simulink model "lc_state_fb_obs_estStatesR"  (R2019a)
settings: Solver=VariableStepAuto  StartTime=0.0  StopTime=60  RelTol=1e-3
values from neighbouring files (symbols this model uses):
  A = [-2 -timeHeadway 0]    [Controller.m]    (also in SimulinkScenario.m = [1 0 0;beta1 1 0; beta0 beta1 1; 0 beta0 beta1; 0 0 beta0])
  B = [0; b1; 0; b2]    [SimulinkScenario.m]
  C = [1 timeHeadway 0; 0 1 timeHeadway; 0 0 1]    [Controller.m]    (also in SimulinkScenario.m = [1 0 0 0])
  Cf = 12e3    (= 12000)    [sim_parameters.m]
  Cr = 11e3    (= 11000)    [sim_parameters.m]
  Iz = 4000    [sim_parameters.m]
  K = A\z    [SimulinkScenario.m]
  L = place(A', C', poles*3)'    [SimulinkScenario.m]
  lf = 1.4    [sim_parameters.m]
  lr = 1.6    [sim_parameters.m]
  maxDelta = 25*pi/180    (= 0.436332312999)    [sim_parameters.m]
  maxDeltaDot = 9.4*pi/180    (= 0.164060949687)    [sim_parameters.m]
  vehMass = 2000    [sim_parameters.m]
  vxRef = 20    [SimulinkScenario.m]
libraries: dspsigops x5, autolibshared x5
settings Model: Creator=Fernando VM  LastModifiedBy=fvall

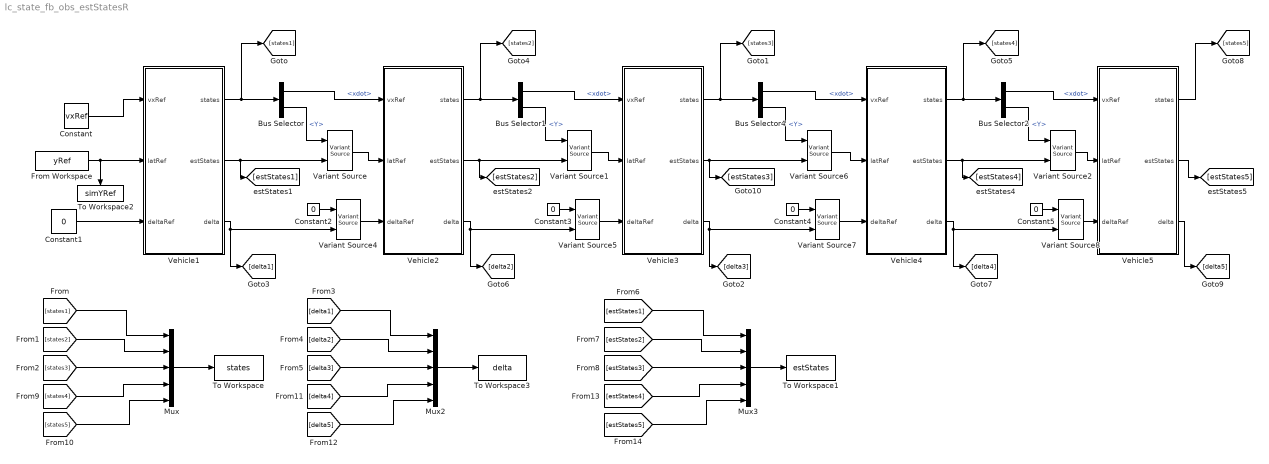
== system lc_state_fb_obs_estStatesR ==
  Bus Selector{,1..2,4} (4 alike) : BusSelector  OutputSignals=xdot,Y
  Constant : Constant  Value=vxRef
  Constant{1..5} (5 alike) : Constant  Value=0
  From Workspace : FromWorkspace  VariableName=yRef  SampleTime=0
  Mux : Mux  Inputs=5
  Mux2 : Mux  Inputs=5
  Mux3 : Mux  Inputs=5
  To Workspace : ToWorkspace  VariableName=states  SampleTime=-1
  To Workspace1 : ToWorkspace  VariableName=estStates  SampleTime=-1
  To Workspace2 : ToWorkspace  VariableName=simYRef  SampleTime=-1
  To Workspace3 : ToWorkspace  VariableName=delta  SampleTime=-1
  Variant Source{,1..2,4..8} (8 alike) : VariantSource
  Vehicle1 : Subsystem  mask{maxDelta=maxDelta, maxDeltaDot=maxDeltaDot, m=vehMass, a=lf, b=lr, Cy_f=Cr, Cy_r=Cf, Izz=Iz, X_o=38.84, initVel=20, sysMatrix=A, inputMatrix=B, C=C, feedbackGain=K, observerGain=L, inputTau=0}
      mask prompts: maxDelta "Max Delta"; maxDeltaDot "Max Delta Variation"; m "autoblks_shared:autoblkVehBody3DofLat:blkPrm_m"; a "autoblks_shared:autoblkVehBody3DofLat:blkPrm_a"; b "autoblks_shared:autoblkVehBody3DofLat:blkPrm_b"; Cy_f "autoblks_shared:autoblkVehBody3DofLat:blkPrm_Cy_f"; Cy_r "autoblks_shared:autoblkVehBody3DofLat:blkPrm_Cy_r"; Izz "autoblks_shared:autoblkVehBody3DofLat:blkPrm_Izz"; X_o "autoblks_shared:autoblkVehBody3DofLat:blkPrm_X_o"; initVel "Initial Long Velocity"; sysMatrix "A"; inputMatrix "B"; feedbackGain "State Feedback Gain Vector"; observerGain "Observer Gain"; inputTau "Input filter time constant"
      mask TypeOptions m: Vehicle Body 3DOF Single Track/m
      mask TypeOptions a: Vehicle Body 3DOF Single Track/a
      mask TypeOptions b: Vehicle Body 3DOF Single Track/b
      mask TypeOptions Cy_f: Vehicle Body 3DOF Single Track/Cy_f
      mask TypeOptions Cy_r: Vehicle Body 3DOF Single Track/Cy_r
      mask TypeOptions Izz: Vehicle Body 3DOF Single Track/Izz
      mask TypeOptions X_o: Vehicle Body 3DOF Single Track/X_o
      mask DialogControl ParameterGroupVar Prompt: Vehicle Parameters
      mask DialogControl m Prompt: Vehicle mass, m [kg]:
      mask DialogControl a Prompt: Longitudinal distance from center of mass to front axle, a [m]:
      mask DialogControl b Prompt: Longitudinal distance from center of mass to rear axle, b [m]:
      mask DialogControl Cy_f Prompt: Front tire corner stiffness, Cy_f [N/rad]:
      mask DialogControl Cy_r Prompt: Rear tire axle corner stiffness, Cy_r [N/rad]:
      mask DialogControl Izz Prompt: Yaw polar inertia, Izz [kg*m^2]:
      mask DialogControl Container6 Prompt: Initial Conditions
      mask DialogControl X_o Prompt: Initial inertial frame longitudinal position, X_o [m]:
      mask DialogControl Container3 Prompt: Linear Model
      mask DialogControl Container5 Prompt: Controller
  Vehicle2 : Subsystem  mask{maxDelta=maxDelta, maxDeltaDot=maxDeltaDot, m=vehMass, a=lf, b=lr, Cy_f=Cr, Cy_r=Cf, Izz=Iz, X_o=29.13, initVel=20, sysMatrix=A, inputMatrix=B, C=C, feedbackGain=K, observerGain=L, inputTau=0}
      mask prompts: maxDelta "Max Delta"; maxDeltaDot "Max Delta Variation"; m "autoblks_shared:autoblkVehBody3DofLat:blkPrm_m"; a "autoblks_shared:autoblkVehBody3DofLat:blkPrm_a"; b "autoblks_shared:autoblkVehBody3DofLat:blkPrm_b"; Cy_f "autoblks_shared:autoblkVehBody3DofLat:blkPrm_Cy_f"; Cy_r "autoblks_shared:autoblkVehBody3DofLat:blkPrm_Cy_r"; Izz "autoblks_shared:autoblkVehBody3DofLat:blkPrm_Izz"; X_o "autoblks_shared:autoblkVehBody3DofLat:blkPrm_X_o"; initVel "Initial Long Velocity"; sysMatrix "A"; inputMatrix "B"; feedbackGain "State Feedback Gain Vector"; observerGain "Observer Gain"; inputTau "Input filter time constant"
      mask TypeOptions m: Vehicle Body 3DOF Single Track/m
      mask TypeOptions a: Vehicle Body 3DOF Single Track/a
      mask TypeOptions b: Vehicle Body 3DOF Single Track/b
      mask TypeOptions Cy_f: Vehicle Body 3DOF Single Track/Cy_f
      mask TypeOptions Cy_r: Vehicle Body 3DOF Single Track/Cy_r
      mask TypeOptions Izz: Vehicle Body 3DOF Single Track/Izz
      mask TypeOptions X_o: Vehicle Body 3DOF Single Track/X_o
      mask DialogControl ParameterGroupVar Prompt: Vehicle Parameters
      mask DialogControl m Prompt: Vehicle mass, m [kg]:
      mask DialogControl a Prompt: Longitudinal distance from center of mass to front axle, a [m]:
      mask DialogControl b Prompt: Longitudinal distance from center of mass to rear axle, b [m]:
      mask DialogControl Cy_f Prompt: Front tire corner stiffness, Cy_f [N/rad]:
      mask DialogControl Cy_r Prompt: Rear tire axle corner stiffness, Cy_r [N/rad]:
      mask DialogControl Izz Prompt: Yaw polar inertia, Izz [kg*m^2]:
      mask DialogControl Container6 Prompt: Initial Conditions
      mask DialogControl X_o Prompt: Initial inertial frame longitudinal position, X_o [m]:
      mask DialogControl Container3 Prompt: Linear Model
      mask DialogControl Container5 Prompt: Controller
  Vehicle3 : Subsystem  mask{maxDelta=maxDelta, maxDeltaDot=maxDeltaDot, m=vehMass, a=lf, b=lr, Cy_f=Cr, Cy_r=Cf, Izz=Iz, X_o=19.42, initVel=20, sysMatrix=A, inputMatrix=B, C=C, feedbackGain=K, observerGain=L, inputTau=0}
      mask prompts: maxDelta "Max Delta"; maxDeltaDot "Max Delta Variation"; m "autoblks_shared:autoblkVehBody3DofLat:blkPrm_m"; a "autoblks_shared:autoblkVehBody3DofLat:blkPrm_a"; b "autoblks_shared:autoblkVehBody3DofLat:blkPrm_b"; Cy_f "autoblks_shared:autoblkVehBody3DofLat:blkPrm_Cy_f"; Cy_r "autoblks_shared:autoblkVehBody3DofLat:blkPrm_Cy_r"; Izz "autoblks_shared:autoblkVehBody3DofLat:blkPrm_Izz"; X_o "autoblks_shared:autoblkVehBody3DofLat:blkPrm_X_o"; initVel "Initial Long Velocity"; sysMatrix "A"; inputMatrix "B"; feedbackGain "State Feedback Gain Vector"; observerGain "Observer Gain"; inputTau "Input filter time constant"
      mask TypeOptions m: Vehicle Body 3DOF Single Track/m
      mask TypeOptions a: Vehicle Body 3DOF Single Track/a
      mask TypeOptions b: Vehicle Body 3DOF Single Track/b
      mask TypeOptions Cy_f: Vehicle Body 3DOF Single Track/Cy_f
      mask TypeOptions Cy_r: Vehicle Body 3DOF Single Track/Cy_r
      mask TypeOptions Izz: Vehicle Body 3DOF Single Track/Izz
      mask TypeOptions X_o: Vehicle Body 3DOF Single Track/X_o
      mask DialogControl ParameterGroupVar Prompt: Vehicle Parameters
      mask DialogControl m Prompt: Vehicle mass, m [kg]:
      mask DialogControl a Prompt: Longitudinal distance from center of mass to front axle, a [m]:
      mask DialogControl b Prompt: Longitudinal distance from center of mass to rear axle, b [m]:
      mask DialogControl Cy_f Prompt: Front tire corner stiffness, Cy_f [N/rad]:
      mask DialogControl Cy_r Prompt: Rear tire axle corner stiffness, Cy_r [N/rad]:
      mask DialogControl Izz Prompt: Yaw polar inertia, Izz [kg*m^2]:
      mask DialogControl Container6 Prompt: Initial Conditions
      mask DialogControl X_o Prompt: Initial inertial frame longitudinal position, X_o [m]:
      mask DialogControl Container3 Prompt: Linear Model
      mask DialogControl Container5 Prompt: Controller
  Vehicle4 : Subsystem  mask{maxDelta=maxDelta, maxDeltaDot=maxDeltaDot, m=vehMass, a=lf, b=lr, Cy_f=Cr, Cy_r=Cf, Izz=Iz, X_o=9.71, initVel=20, sysMatrix=A, inputMatrix=B, C=C, feedbackGain=K, observerGain=L, inputTau=0}
      mask prompts: maxDelta "Max Delta"; maxDeltaDot "Max Delta Variation"; m "autoblks_shared:autoblkVehBody3DofLat:blkPrm_m"; a "autoblks_shared:autoblkVehBody3DofLat:blkPrm_a"; b "autoblks_shared:autoblkVehBody3DofLat:blkPrm_b"; Cy_f "autoblks_shared:autoblkVehBody3DofLat:blkPrm_Cy_f"; Cy_r "autoblks_shared:autoblkVehBody3DofLat:blkPrm_Cy_r"; Izz "autoblks_shared:autoblkVehBody3DofLat:blkPrm_Izz"; X_o "autoblks_shared:autoblkVehBody3DofLat:blkPrm_X_o"; initVel "Initial Long Velocity"; sysMatrix "A"; inputMatrix "B"; feedbackGain "State Feedback Gain Vector"; observerGain "Observer Gain"; inputTau "Input filter time constant"
      mask TypeOptions m: Vehicle Body 3DOF Single Track/m
      mask TypeOptions a: Vehicle Body 3DOF Single Track/a
      mask TypeOptions b: Vehicle Body 3DOF Single Track/b
      mask TypeOptions Cy_f: Vehicle Body 3DOF Single Track/Cy_f
      mask TypeOptions Cy_r: Vehicle Body 3DOF Single Track/Cy_r
      mask TypeOptions Izz: Vehicle Body 3DOF Single Track/Izz
      mask TypeOptions X_o: Vehicle Body 3DOF Single Track/X_o
      mask DialogControl ParameterGroupVar Prompt: Vehicle Parameters
      mask DialogControl m Prompt: Vehicle mass, m [kg]:
      mask DialogControl a Prompt: Longitudinal distance from center of mass to front axle, a [m]:
      mask DialogControl b Prompt: Longitudinal distance from center of mass to rear axle, b [m]:
      mask DialogControl Cy_f Prompt: Front tire corner stiffness, Cy_f [N/rad]:
      mask DialogControl Cy_r Prompt: Rear tire axle corner stiffness, Cy_r [N/rad]:
      mask DialogControl Izz Prompt: Yaw polar inertia, Izz [kg*m^2]:
      mask DialogControl Container6 Prompt: Initial Conditions
      mask DialogControl X_o Prompt: Initial inertial frame longitudinal position, X_o [m]:
      mask DialogControl Container3 Prompt: Linear Model
      mask DialogControl Container5 Prompt: Controller
  Vehicle5 : Subsystem  mask{maxDelta=maxDelta, maxDeltaDot=maxDeltaDot, m=vehMass, a=lf, b=lr, Cy_f=Cr, Cy_r=Cf, Izz=Iz, X_o=0, initVel=20, sysMatrix=A, inputMatrix=B, C=C, feedbackGain=K, observerGain=L, inputTau=0}
      mask prompts: maxDelta "Max Delta"; maxDeltaDot "Max Delta Variation"; m "autoblks_shared:autoblkVehBody3DofLat:blkPrm_m"; a "autoblks_shared:autoblkVehBody3DofLat:blkPrm_a"; b "autoblks_shared:autoblkVehBody3DofLat:blkPrm_b"; Cy_f "autoblks_shared:autoblkVehBody3DofLat:blkPrm_Cy_f"; Cy_r "autoblks_shared:autoblkVehBody3DofLat:blkPrm_Cy_r"; Izz "autoblks_shared:autoblkVehBody3DofLat:blkPrm_Izz"; X_o "autoblks_shared:autoblkVehBody3DofLat:blkPrm_X_o"; initVel "Initial Long Velocity"; sysMatrix "A"; inputMatrix "B"; feedbackGain "State Feedback Gain Vector"; observerGain "Observer Gain"; inputTau "Input filter time constant"
      mask TypeOptions m: Vehicle Body 3DOF Single Track/m
      mask TypeOptions a: Vehicle Body 3DOF Single Track/a
      mask TypeOptions b: Vehicle Body 3DOF Single Track/b
      mask TypeOptions Cy_f: Vehicle Body 3DOF Single Track/Cy_f
      mask TypeOptions Cy_r: Vehicle Body 3DOF Single Track/Cy_r
      mask TypeOptions Izz: Vehicle Body 3DOF Single Track/Izz
      mask TypeOptions X_o: Vehicle Body 3DOF Single Track/X_o
      mask DialogControl ParameterGroupVar Prompt: Vehicle Parameters
      mask DialogControl m Prompt: Vehicle mass, m [kg]:
      mask DialogControl a Prompt: Longitudinal distance from center of mass to front axle, a [m]:
      mask DialogControl b Prompt: Longitudinal distance from center of mass to rear axle, b [m]:
      mask DialogControl Cy_f Prompt: Front tire corner stiffness, Cy_f [N/rad]:
      mask DialogControl Cy_r Prompt: Rear tire axle corner stiffness, Cy_r [N/rad]:
      mask DialogControl Izz Prompt: Yaw polar inertia, Izz [kg*m^2]:
      mask DialogControl Container6 Prompt: Initial Conditions
      mask DialogControl X_o Prompt: Initial inertial frame longitudinal position, X_o [m]:
      mask DialogControl Container3 Prompt: Linear Model
      mask DialogControl Container5 Prompt: Controller
  wires:
  From Workspace/1 -> Vehicle1/2(latRef), To Workspace2/1
  Constant/1 -> Vehicle1/1(vxRef)
  Vehicle1/1(states) -> [states1], Bus Selector/1
  Vehicle1/2(estStates) -> [estStates1], Variant Source/2
  Mux/1 -> To Workspace/1
  [states1] -> Mux/1
  [states2] -> Mux/2
  [states3] -> Mux/3
  Vehicle1/3(delta) -> [delta1], Variant Source4/2
  [states4] -> Mux/4
  [states5] -> Mux/5
  [delta4] -> Mux2/4
  [delta5] -> Mux2/5
  [delta1] -> Mux2/1
  [delta2] -> Mux2/2
  [delta3] -> Mux2/3
  Mux2/1 -> To Workspace3/1
  [estStates4] -> Mux3/4
  [estStates5] -> Mux3/5
  [estStates1] -> Mux3/1
  [estStates2] -> Mux3/2
  [estStates3] -> Mux3/3
  Mux3/1 -> To Workspace1/1
  Bus Selector/2 -> Variant Source/1  "<Y>"
  Bus Selector/1 -> Vehicle2/1(vxRef)  "<xdot>"
  Variant Source/1 -> Vehicle2/2(latRef)
  Constant1/1 -> Vehicle1/3(deltaRef)
  Constant2/1 -> Variant Source4/1
  Variant Source4/1 -> Vehicle2/3(deltaRef)
  Bus Selector1/2 -> Variant Source1/1  "<Y>"
  Vehicle2/2(estStates) -> [estStates2], Variant Source1/2
  Vehicle2/3(delta) -> [delta2], Variant Source5/2
  Variant Source5/1 -> Vehicle3/3(deltaRef)
  Vehicle2/1(states) -> [states2], Bus Selector1/1
  Bus Selector1/1 -> Vehicle3/1(vxRef)  "<xdot>"
  Variant Source1/1 -> Vehicle3/2(latRef)
  Constant3/1 -> Variant Source5/1
  Constant4/1 -> Variant Source7/1
  Vehicle3/2(estStates) -> Variant Source6/2, [estStates3]
  Bus Selector4/2 -> Variant Source6/1  "<Y>"
  Vehicle3/3(delta) -> [delta3], Variant Source7/2
  Vehicle3/1(states) -> [states3], Bus Selector4/1
  Constant5/1 -> Variant Source8/1
  Vehicle4/2(estStates) -> [estStates4], Variant Source2/2
  Bus Selector2/2 -> Variant Source2/1  "<Y>"
  Vehicle4/3(delta) -> [delta4], Variant Source8/2
  Vehicle4/1(states) -> [states4], Bus Selector2/1
  Variant Source7/1 -> Vehicle4/3(deltaRef)
  Variant Source6/1 -> Vehicle4/2(latRef)
  Vehicle5/2(estStates) -> [estStates5]
  Vehicle5/3(delta) -> [delta5]
  Vehicle5/1(states) -> [states5]
  Variant Source8/1 -> Vehicle5/3(deltaRef)
  Variant Source2/1 -> Vehicle5/2(latRef)
  Bus Selector2/1 -> Vehicle5/1(vxRef)  "<xdot>"
  Bus Selector4/1 -> Vehicle4/1(vxRef)  "<xdot>"

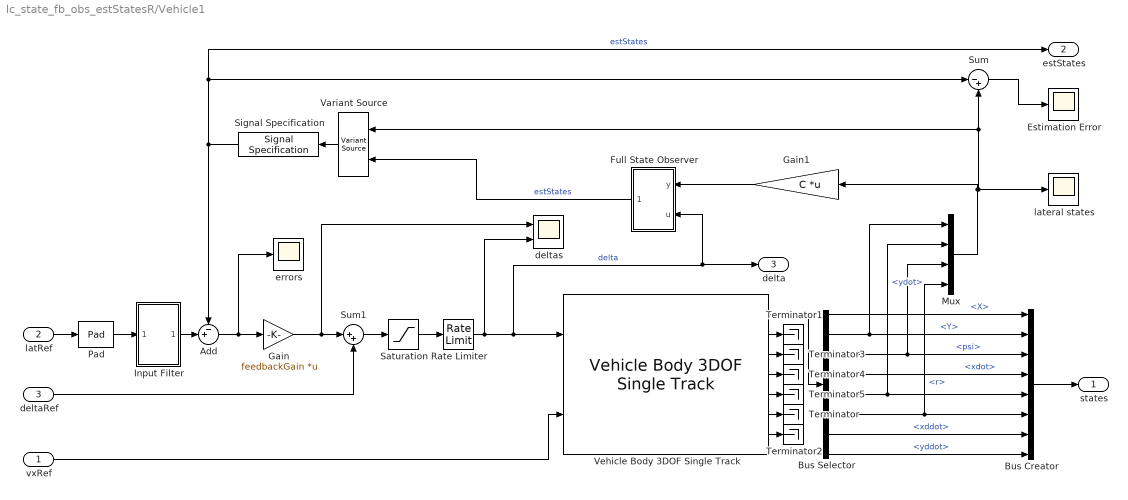
== system lc_state_fb_obs_estStatesR/Vehicle1 ==
  vxRef : Inport
  latRef : Inport  Port=2
  deltaRef : Inport  Port=3
  Add : Sum  Inputs=-+|
  Bus Creator : BusCreator  Inputs=8
  Bus Selector : BusSelector  OutputSignals=InertFrm.Cg.Disp.X,InertFrm.Cg.Disp.Y,InertFrm.Cg.Ang.psi,BdyFrm.Cg.Vel.xdot,BdyFrm.Cg.Vel.ydot,BdyFrm.Cg.AngVel.r,BdyFrm.Cg.Acc.xddot,BdyFrm.Cg.Acc.yddot
  Estimation Error : Scope
  Full State Observer : Subsystem
  Gain : Gain  Gain=feedbackGain  Multiplication=Matrix(K*u)
  Gain1 : Gain  Gain=C  Multiplication=Matrix(K*u)
  Input Filter : Subsystem
  Mux : Mux
  Pad : dspsigops/Pad  padAlong=Columns  dimsToPad=1  valSrc=Specify via dialog  padVal=0  spec=Output size  padNumOutRowsSpecMethod=User-specified  numOutRows=4  padNumOutColsSpecMethod=User-specified  numOutCols=1  isVarDimsMode=off  padBeginning=0  padEnd=0  outSizeMode=User-specified  outSize=1  padSigAt=End  trunc_flag=None  roundingMode=Floor  overflowMode=off  truncOrWrapMode=Truncate  wrap_flag=None
      settings: SourceProductName=DSP System Toolbox  SourceProductBaseCode=DS
  Rate Limiter : RateLimiter  RisingSlewLimit=maxDeltaDot  FallingSlewLimit=-maxDeltaDot  SampleTimeMode=inherited
  Saturation : Saturate  UpperLimit=maxDelta  LowerLimit=-maxDelta
  Signal Specification : SignalSpecification  Dimensions=[4 1]
  Sum : Sum  Inputs=|-+
  Sum1 : Sum  Inputs=|++
  Terminator{,1..5} (6 alike) : Terminator
  Variant Source : VariantSource
  Vehicle Body 3DOF Single Track : autolibshared/Vehicle Body 3DOF Single Track  trackMode=Single (bicycle)  inputMode=External longitudinal velocity  frontSteerMode=on  rearSteerMode=off  windMode=off  muMode=off  extFMode=off  extMMode=off  extXo=off  extpsio=off  extxdoto=off  extro=off  extYo=off  extTamb=off  extydoto=off  aMode=2  NF=2  NR=2  m=m  a=a  b=b  h=0.35  X_o=X_o  xdot_o=0  CalphaMode=off  sigmaMode=on  d=0  w=[1.4,1.4]  Cy_f=Cy_f  Cy_r=Cy_r  sigma_f=.1  sigma_r=.1  alpha_f_brk=[-.1 .1]  Cy_f_data=[-9e3 9e3]  alpha_r_brk=[-.1 .1]  Cy_r_data=[-9e3 9e3]  Y_o=0  ydot_o=0  Izz=Izz  psi_o=0  r_o=0  Af=2  Cd=.3  Cl=.1  Cpm=.1  beta_w=[0:0.01:0.3]  Cs=[0:0.03:0.9]  Cym=[0:0.01:0.3]  Pabs=101325  Tair=273  g=9.81  mu=1  xdot_tol=.01  Fznom=5000  Fxtire_sat=7e4  Fytire_sat=7e4  longOff=0  latOff=0  vertOff=0  wrapAng=off
      settings: SourceProductName=Powertrain Blockset  SourceProductBaseCode=PW
  deltas : Scope  NumInputPorts=2
  errors : Scope
  lateral states : Scope
  states : Outport
  estStates : Outport  Port=2
  delta : Outport  Port=3
  wires:
  Add/1 -> errors/1, Gain/1
  Gain/1 -> Sum1/1, deltas/1
  Vehicle Body 3DOF Single Track/1 -> Bus Selector/1
  Bus Selector/2 -> Bus Creator/2, Mux/1  "<Y>"
  Saturation/1 -> Rate Limiter/1
  vxRef/1 -> Vehicle Body 3DOF Single Track/2
  Sum/1 -> Estimation Error/1
  latRef/1 -> Pad/1
  Input Filter/1(Out1) -> Add/2
  Vehicle Body 3DOF Single Track/2 -> Terminator1/1
  Vehicle Body 3DOF Single Track/6 -> Terminator/1
  Vehicle Body 3DOF Single Track/7 -> Terminator2/1
  Bus Selector/5 -> Mux/2, Bus Creator/5  "<ydot>"
  Bus Selector/3 -> Bus Creator/3, Mux/3  "<psi>"
  Bus Selector/6 -> Bus Creator/6, Mux/4  "<r>"
  Vehicle Body 3DOF Single Track/3 -> Terminator3/1
  Vehicle Body 3DOF Single Track/4 -> Terminator4/1
  Vehicle Body 3DOF Single Track/5 -> Terminator5/1
  Bus Creator/1 -> states/1
  Bus Selector/1 -> Bus Creator/1  "<X>"
  Bus Selector/4 -> Bus Creator/4  "<xdot>"
  Bus Selector/7 -> Bus Creator/7  "<xddot>"
  Bus Selector/8 -> Bus Creator/8  "<yddot>"
  Variant Source/1 -> Signal Specification/1
  Gain1/1 -> Full State Observer/1(y)
  Mux/1 -> Gain1/1, Variant Source/1, Sum/2, lateral states/1
  Full State Observer/1(xhat) -> Variant Source/2  "estStates"
  Rate Limiter/1 -> Vehicle Body 3DOF Single Track/1, Full State Observer/2(u), delta/1, deltas/2  "delta"
  Signal Specification/1 -> estStates/1, Sum/1, Add/1  "estStates"
  Pad/1 -> Input Filter/1(In1)
  Sum1/1 -> Saturation/1
  deltaRef/1 -> Sum1/2

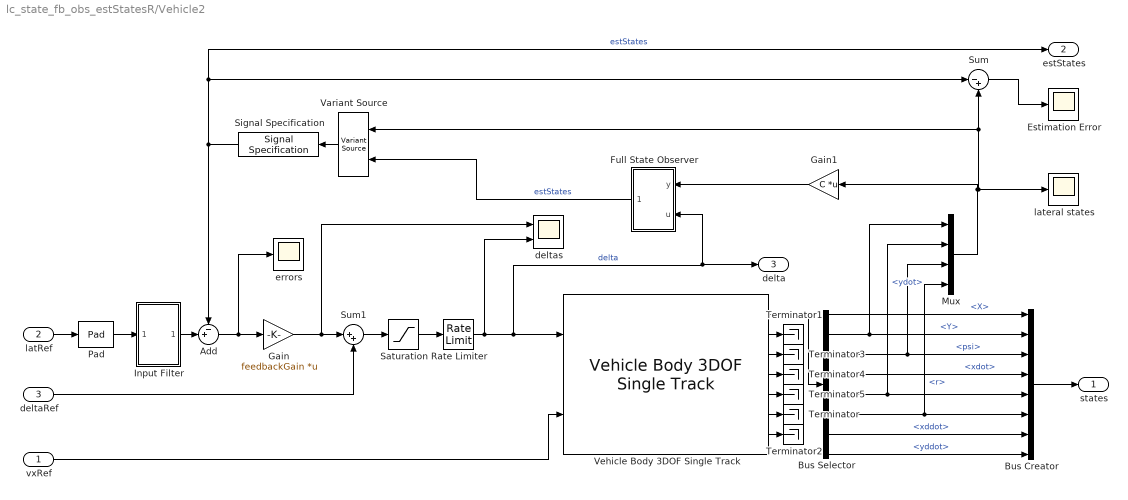
== system lc_state_fb_obs_estStatesR/Vehicle2 ==
  vxRef : Inport
  latRef : Inport  Port=2
  deltaRef : Inport  Port=3
  Add : Sum  Inputs=-+|
  Bus Creator : BusCreator  Inputs=8
  Bus Selector : BusSelector  OutputSignals=InertFrm.Cg.Disp.X,InertFrm.Cg.Disp.Y,InertFrm.Cg.Ang.psi,BdyFrm.Cg.Vel.xdot,BdyFrm.Cg.Vel.ydot,BdyFrm.Cg.AngVel.r,BdyFrm.Cg.Acc.xddot,BdyFrm.Cg.Acc.yddot
  Estimation Error : Scope
  Full State Observer : Subsystem
  Gain : Gain  Gain=feedbackGain  Multiplication=Matrix(K*u)
  Gain1 : Gain  Gain=C  Multiplication=Matrix(K*u)
  Input Filter : Subsystem
  Mux : Mux
  Pad : dspsigops/Pad  padAlong=Columns  dimsToPad=1  valSrc=Specify via dialog  padVal=0  spec=Output size  padNumOutRowsSpecMethod=User-specified  numOutRows=4  padNumOutColsSpecMethod=User-specified  numOutCols=1  isVarDimsMode=off  padBeginning=0  padEnd=0  outSizeMode=User-specified  outSize=1  padSigAt=End  trunc_flag=None  roundingMode=Floor  overflowMode=off  truncOrWrapMode=Truncate  wrap_flag=None
      settings: SourceProductName=DSP System Toolbox  SourceProductBaseCode=DS
  Rate Limiter : RateLimiter  RisingSlewLimit=maxDeltaDot  FallingSlewLimit=-maxDeltaDot  SampleTimeMode=inherited
  Saturation : Saturate  UpperLimit=maxDelta  LowerLimit=-maxDelta
  Signal Specification : SignalSpecification  Dimensions=[4 1]
  Sum : Sum  Inputs=|-+
  Sum1 : Sum  Inputs=|++
  Terminator{,1..5} (6 alike) : Terminator
  Variant Source : VariantSource
  Vehicle Body 3DOF Single Track : autolibshared/Vehicle Body 3DOF Single Track  trackMode=Single (bicycle)  inputMode=External longitudinal velocity  frontSteerMode=on  rearSteerMode=off  windMode=off  muMode=off  extFMode=off  extMMode=off  extXo=off  extpsio=off  extxdoto=off  extro=off  extYo=off  extTamb=off  extydoto=off  aMode=2  NF=2  NR=2  m=m  a=a  b=b  h=0.35  X_o=X_o  xdot_o=0  CalphaMode=off  sigmaMode=on  d=0  w=[1.4,1.4]  Cy_f=Cy_f  Cy_r=Cy_r  sigma_f=.1  sigma_r=.1  alpha_f_brk=[-.1 .1]  Cy_f_data=[-9e3 9e3]  alpha_r_brk=[-.1 .1]  Cy_r_data=[-9e3 9e3]  Y_o=0  ydot_o=0  Izz=Izz  psi_o=0  r_o=0  Af=2  Cd=.3  Cl=.1  Cpm=.1  beta_w=[0:0.01:0.3]  Cs=[0:0.03:0.9]  Cym=[0:0.01:0.3]  Pabs=101325  Tair=273  g=9.81  mu=1  xdot_tol=.01  Fznom=5000  Fxtire_sat=7e4  Fytire_sat=7e4  longOff=0  latOff=0  vertOff=0  wrapAng=off
      settings: SourceProductName=Powertrain Blockset  SourceProductBaseCode=PW
  deltas : Scope  NumInputPorts=2
  errors : Scope
  lateral states : Scope
  states : Outport
  estStates : Outport  Port=2
  delta : Outport  Port=3
  wires:
  Add/1 -> errors/1, Gain/1
  Gain/1 -> Sum1/1, deltas/1
  Vehicle Body 3DOF Single Track/1 -> Bus Selector/1
  Bus Selector/2 -> Bus Creator/2, Mux/1  "<Y>"
  Saturation/1 -> Rate Limiter/1
  vxRef/1 -> Vehicle Body 3DOF Single Track/2
  Sum/1 -> Estimation Error/1
  latRef/1 -> Pad/1
  Input Filter/1(Out1) -> Add/2
  Vehicle Body 3DOF Single Track/2 -> Terminator1/1
  Vehicle Body 3DOF Single Track/6 -> Terminator/1
  Vehicle Body 3DOF Single Track/7 -> Terminator2/1
  Bus Selector/5 -> Mux/2, Bus Creator/5  "<ydot>"
  Bus Selector/3 -> Bus Creator/3, Mux/3  "<psi>"
  Bus Selector/6 -> Bus Creator/6, Mux/4  "<r>"
  Vehicle Body 3DOF Single Track/3 -> Terminator3/1
  Vehicle Body 3DOF Single Track/4 -> Terminator4/1
  Vehicle Body 3DOF Single Track/5 -> Terminator5/1
  Bus Creator/1 -> states/1
  Bus Selector/1 -> Bus Creator/1  "<X>"
  Bus Selector/4 -> Bus Creator/4  "<xdot>"
  Bus Selector/7 -> Bus Creator/7  "<xddot>"
  Bus Selector/8 -> Bus Creator/8  "<yddot>"
  Variant Source/1 -> Signal Specification/1
  Gain1/1 -> Full State Observer/1(y)
  Mux/1 -> Gain1/1, Variant Source/1, Sum/2, lateral states/1
  Full State Observer/1(xhat) -> Variant Source/2  "estStates"
  Rate Limiter/1 -> Vehicle Body 3DOF Single Track/1, Full State Observer/2(u), delta/1, deltas/2  "delta"
  Signal Specification/1 -> estStates/1, Sum/1, Add/1  "estStates"
  Pad/1 -> Input Filter/1(In1)
  Sum1/1 -> Saturation/1
  deltaRef/1 -> Sum1/2

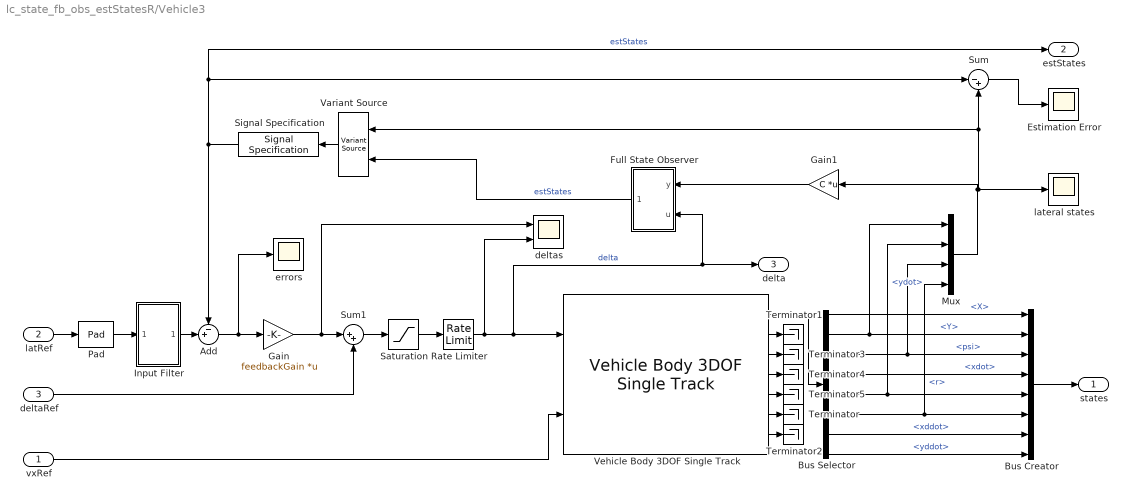
== system lc_state_fb_obs_estStatesR/Vehicle3 ==
  vxRef : Inport
  latRef : Inport  Port=2
  deltaRef : Inport  Port=3
  Add : Sum  Inputs=-+|
  Bus Creator : BusCreator  Inputs=8
  Bus Selector : BusSelector  OutputSignals=InertFrm.Cg.Disp.X,InertFrm.Cg.Disp.Y,InertFrm.Cg.Ang.psi,BdyFrm.Cg.Vel.xdot,BdyFrm.Cg.Vel.ydot,BdyFrm.Cg.AngVel.r,BdyFrm.Cg.Acc.xddot,BdyFrm.Cg.Acc.yddot
  Estimation Error : Scope
  Full State Observer : Subsystem
  Gain : Gain  Gain=feedbackGain  Multiplication=Matrix(K*u)
  Gain1 : Gain  Gain=C  Multiplication=Matrix(K*u)
  Input Filter : Subsystem
  Mux : Mux
  Pad : dspsigops/Pad  padAlong=Columns  dimsToPad=1  valSrc=Specify via dialog  padVal=0  spec=Output size  padNumOutRowsSpecMethod=User-specified  numOutRows=4  padNumOutColsSpecMethod=User-specified  numOutCols=1  isVarDimsMode=off  padBeginning=0  padEnd=0  outSizeMode=User-specified  outSize=1  padSigAt=End  trunc_flag=None  roundingMode=Floor  overflowMode=off  truncOrWrapMode=Truncate  wrap_flag=None
      settings: SourceProductName=DSP System Toolbox  SourceProductBaseCode=DS
  Rate Limiter : RateLimiter  RisingSlewLimit=maxDeltaDot  FallingSlewLimit=-maxDeltaDot  SampleTimeMode=inherited
  Saturation : Saturate  UpperLimit=maxDelta  LowerLimit=-maxDelta
  Signal Specification : SignalSpecification  Dimensions=[4 1]
  Sum : Sum  Inputs=|-+
  Sum1 : Sum  Inputs=|++
  Terminator{,1..5} (6 alike) : Terminator
  Variant Source : VariantSource
  Vehicle Body 3DOF Single Track : autolibshared/Vehicle Body 3DOF Single Track  trackMode=Single (bicycle)  inputMode=External longitudinal velocity  frontSteerMode=on  rearSteerMode=off  windMode=off  muMode=off  extFMode=off  extMMode=off  extXo=off  extpsio=off  extxdoto=off  extro=off  extYo=off  extTamb=off  extydoto=off  aMode=2  NF=2  NR=2  m=m  a=a  b=b  h=0.35  X_o=X_o  xdot_o=0  CalphaMode=off  sigmaMode=on  d=0  w=[1.4,1.4]  Cy_f=Cy_f  Cy_r=Cy_r  sigma_f=.1  sigma_r=.1  alpha_f_brk=[-.1 .1]  Cy_f_data=[-9e3 9e3]  alpha_r_brk=[-.1 .1]  Cy_r_data=[-9e3 9e3]  Y_o=0  ydot_o=0  Izz=Izz  psi_o=0  r_o=0  Af=2  Cd=.3  Cl=.1  Cpm=.1  beta_w=[0:0.01:0.3]  Cs=[0:0.03:0.9]  Cym=[0:0.01:0.3]  Pabs=101325  Tair=273  g=9.81  mu=1  xdot_tol=.01  Fznom=5000  Fxtire_sat=7e4  Fytire_sat=7e4  longOff=0  latOff=0  vertOff=0  wrapAng=off
      settings: SourceProductName=Powertrain Blockset  SourceProductBaseCode=PW
  deltas : Scope  NumInputPorts=2
  errors : Scope
  lateral states : Scope
  states : Outport
  estStates : Outport  Port=2
  delta : Outport  Port=3
  wires:
  Add/1 -> errors/1, Gain/1
  Gain/1 -> Sum1/1, deltas/1
  Vehicle Body 3DOF Single Track/1 -> Bus Selector/1
  Bus Selector/2 -> Bus Creator/2, Mux/1  "<Y>"
  Saturation/1 -> Rate Limiter/1
  vxRef/1 -> Vehicle Body 3DOF Single Track/2
  Sum/1 -> Estimation Error/1
  latRef/1 -> Pad/1
  Input Filter/1(Out1) -> Add/2
  Vehicle Body 3DOF Single Track/2 -> Terminator1/1
  Vehicle Body 3DOF Single Track/6 -> Terminator/1
  Vehicle Body 3DOF Single Track/7 -> Terminator2/1
  Bus Selector/5 -> Mux/2, Bus Creator/5  "<ydot>"
  Bus Selector/3 -> Bus Creator/3, Mux/3  "<psi>"
  Bus Selector/6 -> Bus Creator/6, Mux/4  "<r>"
  Vehicle Body 3DOF Single Track/3 -> Terminator3/1
  Vehicle Body 3DOF Single Track/4 -> Terminator4/1
  Vehicle Body 3DOF Single Track/5 -> Terminator5/1
  Bus Creator/1 -> states/1
  Bus Selector/1 -> Bus Creator/1  "<X>"
  Bus Selector/4 -> Bus Creator/4  "<xdot>"
  Bus Selector/7 -> Bus Creator/7  "<xddot>"
  Bus Selector/8 -> Bus Creator/8  "<yddot>"
  Variant Source/1 -> Signal Specification/1
  Gain1/1 -> Full State Observer/1(y)
  Mux/1 -> Gain1/1, Variant Source/1, Sum/2, lateral states/1
  Full State Observer/1(xhat) -> Variant Source/2  "estStates"
  Rate Limiter/1 -> Vehicle Body 3DOF Single Track/1, Full State Observer/2(u), delta/1, deltas/2  "delta"
  Signal Specification/1 -> estStates/1, Sum/1, Add/1  "estStates"
  Pad/1 -> Input Filter/1(In1)
  Sum1/1 -> Saturation/1
  deltaRef/1 -> Sum1/2

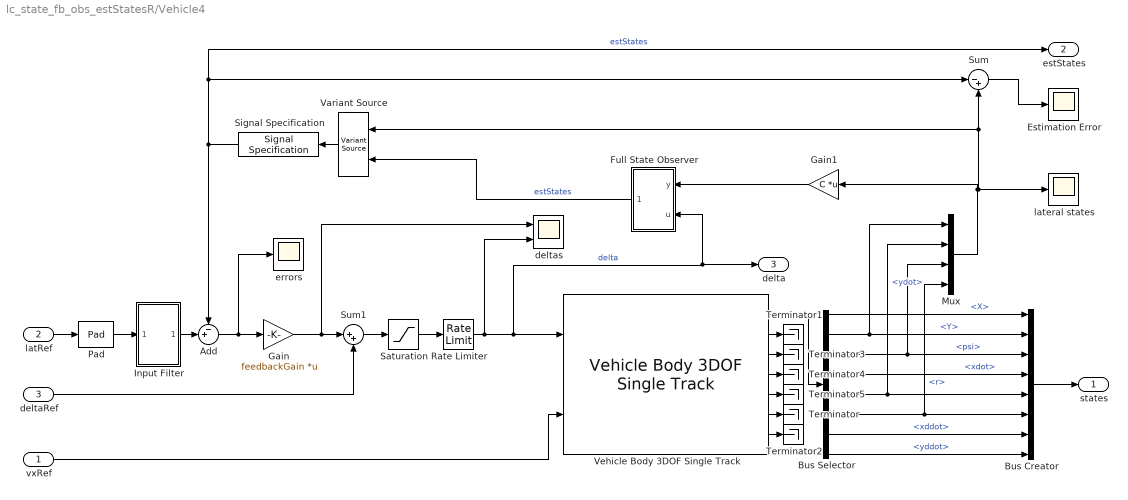
== system lc_state_fb_obs_estStatesR/Vehicle4 ==
  vxRef : Inport
  latRef : Inport  Port=2
  deltaRef : Inport  Port=3
  Add : Sum  Inputs=-+|
  Bus Creator : BusCreator  Inputs=8
  Bus Selector : BusSelector  OutputSignals=InertFrm.Cg.Disp.X,InertFrm.Cg.Disp.Y,InertFrm.Cg.Ang.psi,BdyFrm.Cg.Vel.xdot,BdyFrm.Cg.Vel.ydot,BdyFrm.Cg.AngVel.r,BdyFrm.Cg.Acc.xddot,BdyFrm.Cg.Acc.yddot
  Estimation Error : Scope
  Full State Observer : Subsystem
  Gain : Gain  Gain=feedbackGain  Multiplication=Matrix(K*u)
  Gain1 : Gain  Gain=C  Multiplication=Matrix(K*u)
  Input Filter : Subsystem
  Mux : Mux
  Pad : dspsigops/Pad  padAlong=Columns  dimsToPad=1  valSrc=Specify via dialog  padVal=0  spec=Output size  padNumOutRowsSpecMethod=User-specified  numOutRows=4  padNumOutColsSpecMethod=User-specified  numOutCols=1  isVarDimsMode=off  padBeginning=0  padEnd=0  outSizeMode=User-specified  outSize=1  padSigAt=End  trunc_flag=None  roundingMode=Floor  overflowMode=off  truncOrWrapMode=Truncate  wrap_flag=None
      settings: SourceProductName=DSP System Toolbox  SourceProductBaseCode=DS
  Rate Limiter : RateLimiter  RisingSlewLimit=maxDeltaDot  FallingSlewLimit=-maxDeltaDot  SampleTimeMode=inherited
  Saturation : Saturate  UpperLimit=maxDelta  LowerLimit=-maxDelta
  Signal Specification : SignalSpecification  Dimensions=[4 1]
  Sum : Sum  Inputs=|-+
  Sum1 : Sum  Inputs=|++
  Terminator{,1..5} (6 alike) : Terminator
  Variant Source : VariantSource
  Vehicle Body 3DOF Single Track : autolibshared/Vehicle Body 3DOF Single Track  trackMode=Single (bicycle)  inputMode=External longitudinal velocity  frontSteerMode=on  rearSteerMode=off  windMode=off  muMode=off  extFMode=off  extMMode=off  extXo=off  extpsio=off  extxdoto=off  extro=off  extYo=off  extTamb=off  extydoto=off  aMode=2  NF=2  NR=2  m=m  a=a  b=b  h=0.35  X_o=X_o  xdot_o=0  CalphaMode=off  sigmaMode=on  d=0  w=[1.4,1.4]  Cy_f=Cy_f  Cy_r=Cy_r  sigma_f=.1  sigma_r=.1  alpha_f_brk=[-.1 .1]  Cy_f_data=[-9e3 9e3]  alpha_r_brk=[-.1 .1]  Cy_r_data=[-9e3 9e3]  Y_o=0  ydot_o=0  Izz=Izz  psi_o=0  r_o=0  Af=2  Cd=.3  Cl=.1  Cpm=.1  beta_w=[0:0.01:0.3]  Cs=[0:0.03:0.9]  Cym=[0:0.01:0.3]  Pabs=101325  Tair=273  g=9.81  mu=1  xdot_tol=.01  Fznom=5000  Fxtire_sat=7e4  Fytire_sat=7e4  longOff=0  latOff=0  vertOff=0  wrapAng=off
      settings: SourceProductName=Powertrain Blockset  SourceProductBaseCode=PW
  deltas : Scope  NumInputPorts=2
  errors : Scope
  lateral states : Scope
  states : Outport
  estStates : Outport  Port=2
  delta : Outport  Port=3
  wires:
  Add/1 -> errors/1, Gain/1
  Gain/1 -> Sum1/1, deltas/1
  Vehicle Body 3DOF Single Track/1 -> Bus Selector/1
  Bus Selector/2 -> Bus Creator/2, Mux/1  "<Y>"
  Saturation/1 -> Rate Limiter/1
  vxRef/1 -> Vehicle Body 3DOF Single Track/2
  Sum/1 -> Estimation Error/1
  latRef/1 -> Pad/1
  Input Filter/1(Out1) -> Add/2
  Vehicle Body 3DOF Single Track/2 -> Terminator1/1
  Vehicle Body 3DOF Single Track/6 -> Terminator/1
  Vehicle Body 3DOF Single Track/7 -> Terminator2/1
  Bus Selector/5 -> Mux/2, Bus Creator/5  "<ydot>"
  Bus Selector/3 -> Bus Creator/3, Mux/3  "<psi>"
  Bus Selector/6 -> Bus Creator/6, Mux/4  "<r>"
  Vehicle Body 3DOF Single Track/3 -> Terminator3/1
  Vehicle Body 3DOF Single Track/4 -> Terminator4/1
  Vehicle Body 3DOF Single Track/5 -> Terminator5/1
  Bus Creator/1 -> states/1
  Bus Selector/1 -> Bus Creator/1  "<X>"
  Bus Selector/4 -> Bus Creator/4  "<xdot>"
  Bus Selector/7 -> Bus Creator/7  "<xddot>"
  Bus Selector/8 -> Bus Creator/8  "<yddot>"
  Variant Source/1 -> Signal Specification/1
  Gain1/1 -> Full State Observer/1(y)
  Mux/1 -> Gain1/1, Variant Source/1, Sum/2, lateral states/1
  Full State Observer/1(xhat) -> Variant Source/2  "estStates"
  Rate Limiter/1 -> Vehicle Body 3DOF Single Track/1, Full State Observer/2(u), delta/1, deltas/2  "delta"
  Signal Specification/1 -> estStates/1, Sum/1, Add/1  "estStates"
  Pad/1 -> Input Filter/1(In1)
  Sum1/1 -> Saturation/1
  deltaRef/1 -> Sum1/2

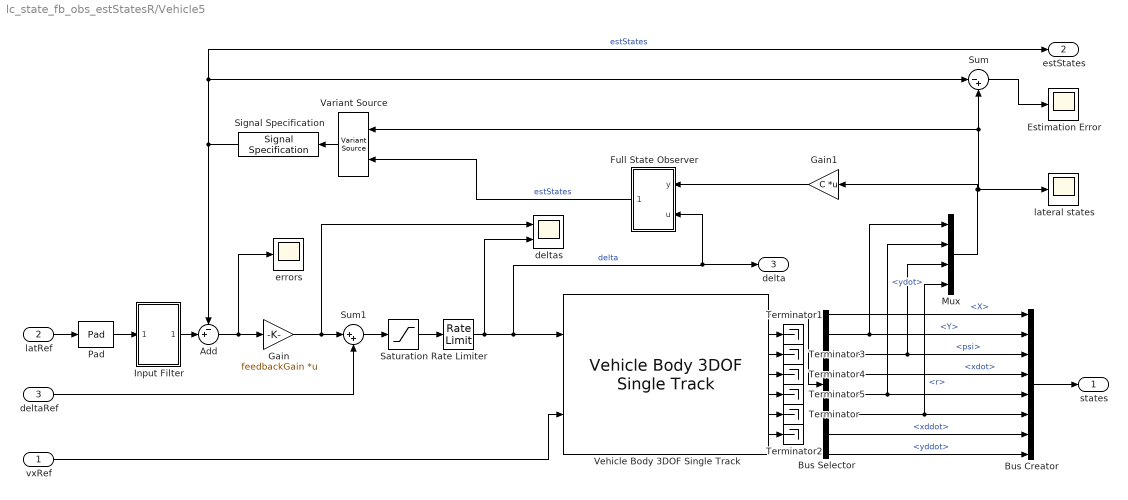
== system lc_state_fb_obs_estStatesR/Vehicle5 ==
  vxRef : Inport
  latRef : Inport  Port=2
  deltaRef : Inport  Port=3
  Add : Sum  Inputs=-+|
  Bus Creator : BusCreator  Inputs=8
  Bus Selector : BusSelector  OutputSignals=InertFrm.Cg.Disp.X,InertFrm.Cg.Disp.Y,InertFrm.Cg.Ang.psi,BdyFrm.Cg.Vel.xdot,BdyFrm.Cg.Vel.ydot,BdyFrm.Cg.AngVel.r,BdyFrm.Cg.Acc.xddot,BdyFrm.Cg.Acc.yddot
  Estimation Error : Scope
  Full State Observer : Subsystem
  Gain : Gain  Gain=feedbackGain  Multiplication=Matrix(K*u)
  Gain1 : Gain  Gain=C  Multiplication=Matrix(K*u)
  Input Filter : Subsystem
  Mux : Mux
  Pad : dspsigops/Pad  padAlong=Columns  dimsToPad=1  valSrc=Specify via dialog  padVal=0  spec=Output size  padNumOutRowsSpecMethod=User-specified  numOutRows=4  padNumOutColsSpecMethod=User-specified  numOutCols=1  isVarDimsMode=off  padBeginning=0  padEnd=0  outSizeMode=User-specified  outSize=1  padSigAt=End  trunc_flag=None  roundingMode=Floor  overflowMode=off  truncOrWrapMode=Truncate  wrap_flag=None
      settings: SourceProductName=DSP System Toolbox  SourceProductBaseCode=DS
  Rate Limiter : RateLimiter  RisingSlewLimit=maxDeltaDot  FallingSlewLimit=-maxDeltaDot  SampleTimeMode=inherited
  Saturation : Saturate  UpperLimit=maxDelta  LowerLimit=-maxDelta
  Signal Specification : SignalSpecification  Dimensions=[4 1]
  Sum : Sum  Inputs=|-+
  Sum1 : Sum  Inputs=|++
  Terminator{,1..5} (6 alike) : Terminator
  Variant Source : VariantSource
  Vehicle Body 3DOF Single Track : autolibshared/Vehicle Body 3DOF Single Track  trackMode=Single (bicycle)  inputMode=External longitudinal velocity  frontSteerMode=on  rearSteerMode=off  windMode=off  muMode=off  extFMode=off  extMMode=off  extXo=off  extpsio=off  extxdoto=off  extro=off  extYo=off  extTamb=off  extydoto=off  aMode=2  NF=2  NR=2  m=m  a=a  b=b  h=0.35  X_o=X_o  xdot_o=0  CalphaMode=off  sigmaMode=on  d=0  w=[1.4,1.4]  Cy_f=Cy_f  Cy_r=Cy_r  sigma_f=.1  sigma_r=.1  alpha_f_brk=[-.1 .1]  Cy_f_data=[-9e3 9e3]  alpha_r_brk=[-.1 .1]  Cy_r_data=[-9e3 9e3]  Y_o=0  ydot_o=0  Izz=Izz  psi_o=0  r_o=0  Af=2  Cd=.3  Cl=.1  Cpm=.1  beta_w=[0:0.01:0.3]  Cs=[0:0.03:0.9]  Cym=[0:0.01:0.3]  Pabs=101325  Tair=273  g=9.81  mu=1  xdot_tol=.01  Fznom=5000  Fxtire_sat=7e4  Fytire_sat=7e4  longOff=0  latOff=0  vertOff=0  wrapAng=off
      settings: SourceProductName=Powertrain Blockset  SourceProductBaseCode=PW
  deltas : Scope  NumInputPorts=2
  errors : Scope
  lateral states : Scope
  states : Outport
  estStates : Outport  Port=2
  delta : Outport  Port=3
  wires:
  Add/1 -> errors/1, Gain/1
  Gain/1 -> Sum1/1, deltas/1
  Vehicle Body 3DOF Single Track/1 -> Bus Selector/1
  Bus Selector/2 -> Bus Creator/2, Mux/1  "<Y>"
  Saturation/1 -> Rate Limiter/1
  vxRef/1 -> Vehicle Body 3DOF Single Track/2
  Sum/1 -> Estimation Error/1
  latRef/1 -> Pad/1
  Input Filter/1(Out1) -> Add/2
  Vehicle Body 3DOF Single Track/2 -> Terminator1/1
  Vehicle Body 3DOF Single Track/6 -> Terminator/1
  Vehicle Body 3DOF Single Track/7 -> Terminator2/1
  Bus Selector/5 -> Mux/2, Bus Creator/5  "<ydot>"
  Bus Selector/3 -> Bus Creator/3, Mux/3  "<psi>"
  Bus Selector/6 -> Bus Creator/6, Mux/4  "<r>"
  Vehicle Body 3DOF Single Track/3 -> Terminator3/1
  Vehicle Body 3DOF Single Track/4 -> Terminator4/1
  Vehicle Body 3DOF Single Track/5 -> Terminator5/1
  Bus Creator/1 -> states/1
  Bus Selector/1 -> Bus Creator/1  "<X>"
  Bus Selector/4 -> Bus Creator/4  "<xdot>"
  Bus Selector/7 -> Bus Creator/7  "<xddot>"
  Bus Selector/8 -> Bus Creator/8  "<yddot>"
  Variant Source/1 -> Signal Specification/1
  Gain1/1 -> Full State Observer/1(y)
  Mux/1 -> Gain1/1, Variant Source/1, Sum/2, lateral states/1
  Full State Observer/1(xhat) -> Variant Source/2  "estStates"
  Rate Limiter/1 -> Vehicle Body 3DOF Single Track/1, Full State Observer/2(u), delta/1, deltas/2  "delta"
  Signal Specification/1 -> estStates/1, Sum/1, Add/1  "estStates"
  Pad/1 -> Input Filter/1(In1)
  Sum1/1 -> Saturation/1
  deltaRef/1 -> Sum1/2

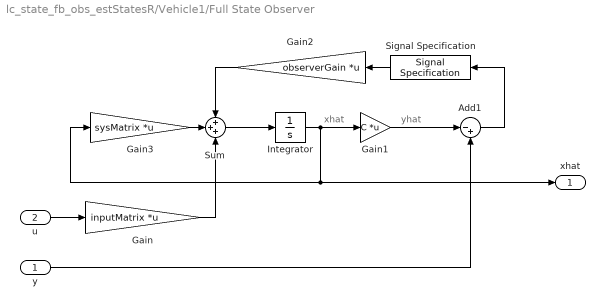
== system lc_state_fb_obs_estStatesR/Vehicle1/Full State Observer ==
  note: xhat
  note: yhat
  y : Inport
  u : Inport  Port=2
  Add1 : Sum  Inputs=|-+
  Gain : Gain  Gain=inputMatrix  Multiplication=Matrix(K*u)
  Gain1 : Gain  Gain=C  Multiplication=Matrix(K*u)
  Gain2 : Gain  Gain=observerGain  Multiplication=Matrix(K*u)
  Gain3 : Gain  Gain=sysMatrix  Multiplication=Matrix(K*u)
  Integrator : Integrator
  Signal Specification : SignalSpecification  Dimensions=[size(C,1) 1]
  Sum : Sum  Inputs=+++
  xhat : Outport
  wires:
  Add1/1 -> Signal Specification/1
  Integrator/1 -> xhat/1, Gain3/1, Gain1/1
  Gain1/1 -> Add1/1
  Sum/1 -> Integrator/1
  y/1 -> Add1/2
  u/1 -> Gain/1
  Gain/1 -> Sum/3
  Gain3/1 -> Sum/2
  Signal Specification/1 -> Gain2/1
  Gain2/1 -> Sum/1

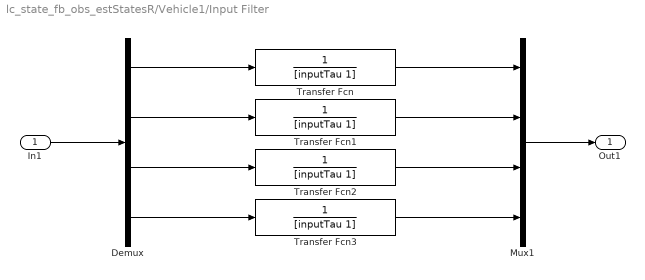
== system lc_state_fb_obs_estStatesR/Vehicle1/Input Filter ==
  In1 : Inport
  Demux : Demux
  Mux1 : Mux
  Transfer Fcn{,1..3} (4 alike) : TransferFcn  Denominator=[inputTau 1]
  Out1 : Outport
  wires:
  Demux/1 -> Transfer Fcn/1
  Demux/2 -> Transfer Fcn1/1
  Demux/3 -> Transfer Fcn2/1
  In1/1 -> Demux/1
  Demux/4 -> Transfer Fcn3/1
  Mux1/1 -> Out1/1
  Transfer Fcn/1 -> Mux1/1
  Transfer Fcn1/1 -> Mux1/2
  Transfer Fcn2/1 -> Mux1/3
  Transfer Fcn3/1 -> Mux1/4

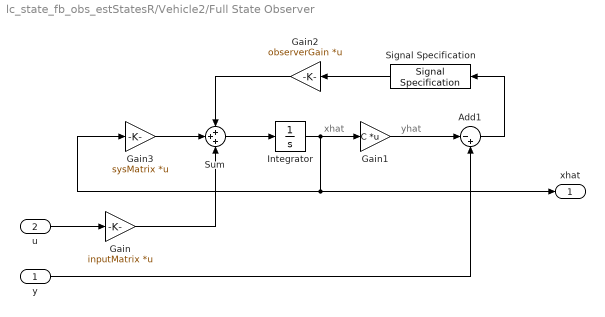
== system lc_state_fb_obs_estStatesR/Vehicle2/Full State Observer ==
  note: xhat
  note: yhat
  y : Inport
  u : Inport  Port=2
  Add1 : Sum  Inputs=|-+
  Gain : Gain  Gain=inputMatrix  Multiplication=Matrix(K*u)
  Gain1 : Gain  Gain=C  Multiplication=Matrix(K*u)
  Gain2 : Gain  Gain=observerGain  Multiplication=Matrix(K*u)
  Gain3 : Gain  Gain=sysMatrix  Multiplication=Matrix(K*u)
  Integrator : Integrator
  Signal Specification : SignalSpecification  Dimensions=[size(C,1) 1]
  Sum : Sum  Inputs=+++
  xhat : Outport
  wires:
  Add1/1 -> Signal Specification/1
  Integrator/1 -> Gain3/1, xhat/1, Gain1/1
  Gain1/1 -> Add1/1
  Sum/1 -> Integrator/1
  y/1 -> Add1/2
  u/1 -> Gain/1
  Gain/1 -> Sum/3
  Gain3/1 -> Sum/2
  Signal Specification/1 -> Gain2/1
  Gain2/1 -> Sum/1

== system lc_state_fb_obs_estStatesR/Vehicle2/Input Filter ==
  In1 : Inport
  Demux : Demux
  Mux1 : Mux
  Transfer Fcn{,1..3} (4 alike) : TransferFcn  Denominator=[inputTau 1]
  Out1 : Outport
  wires:
  Demux/1 -> Transfer Fcn/1
  Demux/2 -> Transfer Fcn1/1
  Demux/3 -> Transfer Fcn2/1
  In1/1 -> Demux/1
  Demux/4 -> Transfer Fcn3/1
  Mux1/1 -> Out1/1
  Transfer Fcn/1 -> Mux1/1
  Transfer Fcn1/1 -> Mux1/2
  Transfer Fcn2/1 -> Mux1/3
  Transfer Fcn3/1 -> Mux1/4

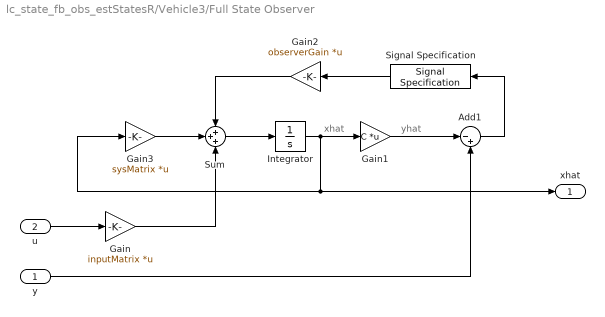
== system lc_state_fb_obs_estStatesR/Vehicle3/Full State Observer ==
  note: xhat
  note: yhat
  y : Inport
  u : Inport  Port=2
  Add1 : Sum  Inputs=|-+
  Gain : Gain  Gain=inputMatrix  Multiplication=Matrix(K*u)
  Gain1 : Gain  Gain=C  Multiplication=Matrix(K*u)
  Gain2 : Gain  Gain=observerGain  Multiplication=Matrix(K*u)
  Gain3 : Gain  Gain=sysMatrix  Multiplication=Matrix(K*u)
  Integrator : Integrator
  Signal Specification : SignalSpecification  Dimensions=[size(C,1) 1]
  Sum : Sum  Inputs=+++
  xhat : Outport
  wires:
  Add1/1 -> Signal Specification/1
  Integrator/1 -> Gain3/1, xhat/1, Gain1/1
  Gain1/1 -> Add1/1
  Sum/1 -> Integrator/1
  y/1 -> Add1/2
  u/1 -> Gain/1
  Gain/1 -> Sum/3
  Gain3/1 -> Sum/2
  Signal Specification/1 -> Gain2/1
  Gain2/1 -> Sum/1

== system lc_state_fb_obs_estStatesR/Vehicle3/Input Filter ==
  In1 : Inport
  Demux : Demux
  Mux1 : Mux
  Transfer Fcn{,1..3} (4 alike) : TransferFcn  Denominator=[inputTau 1]
  Out1 : Outport
  wires:
  Demux/1 -> Transfer Fcn/1
  Demux/2 -> Transfer Fcn1/1
  Demux/3 -> Transfer Fcn2/1
  In1/1 -> Demux/1
  Demux/4 -> Transfer Fcn3/1
  Mux1/1 -> Out1/1
  Transfer Fcn/1 -> Mux1/1
  Transfer Fcn1/1 -> Mux1/2
  Transfer Fcn2/1 -> Mux1/3
  Transfer Fcn3/1 -> Mux1/4

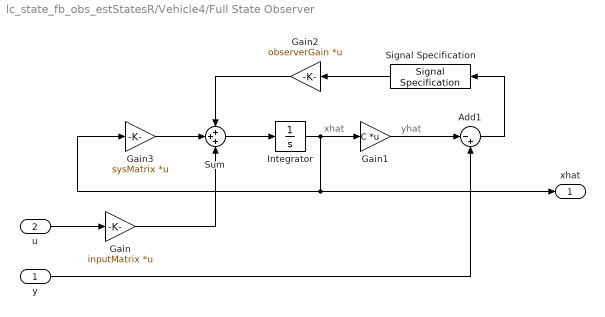
== system lc_state_fb_obs_estStatesR/Vehicle4/Full State Observer ==
  note: xhat
  note: yhat
  y : Inport
  u : Inport  Port=2
  Add1 : Sum  Inputs=|-+
  Gain : Gain  Gain=inputMatrix  Multiplication=Matrix(K*u)
  Gain1 : Gain  Gain=C  Multiplication=Matrix(K*u)
  Gain2 : Gain  Gain=observerGain  Multiplication=Matrix(K*u)
  Gain3 : Gain  Gain=sysMatrix  Multiplication=Matrix(K*u)
  Integrator : Integrator
  Signal Specification : SignalSpecification  Dimensions=[size(C,1) 1]
  Sum : Sum  Inputs=+++
  xhat : Outport
  wires:
  Add1/1 -> Signal Specification/1
  Integrator/1 -> Gain3/1, xhat/1, Gain1/1
  Gain1/1 -> Add1/1
  Sum/1 -> Integrator/1
  y/1 -> Add1/2
  u/1 -> Gain/1
  Gain/1 -> Sum/3
  Gain3/1 -> Sum/2
  Signal Specification/1 -> Gain2/1
  Gain2/1 -> Sum/1

== system lc_state_fb_obs_estStatesR/Vehicle4/Input Filter ==
  In1 : Inport
  Demux : Demux
  Mux1 : Mux
  Transfer Fcn{,1..3} (4 alike) : TransferFcn  Denominator=[inputTau 1]
  Out1 : Outport
  wires:
  Demux/1 -> Transfer Fcn/1
  Demux/2 -> Transfer Fcn1/1
  Demux/3 -> Transfer Fcn2/1
  In1/1 -> Demux/1
  Demux/4 -> Transfer Fcn3/1
  Mux1/1 -> Out1/1
  Transfer Fcn/1 -> Mux1/1
  Transfer Fcn1/1 -> Mux1/2
  Transfer Fcn2/1 -> Mux1/3
  Transfer Fcn3/1 -> Mux1/4

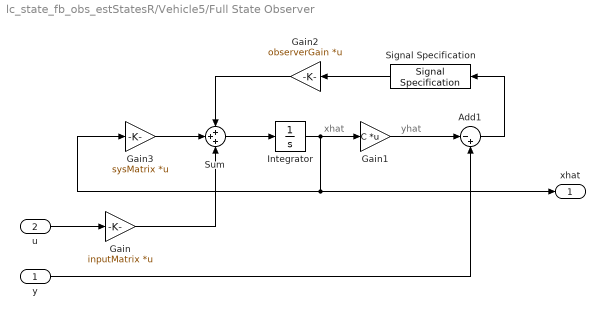
== system lc_state_fb_obs_estStatesR/Vehicle5/Full State Observer ==
  note: xhat
  note: yhat
  y : Inport
  u : Inport  Port=2
  Add1 : Sum  Inputs=|-+
  Gain : Gain  Gain=inputMatrix  Multiplication=Matrix(K*u)
  Gain1 : Gain  Gain=C  Multiplication=Matrix(K*u)
  Gain2 : Gain  Gain=observerGain  Multiplication=Matrix(K*u)
  Gain3 : Gain  Gain=sysMatrix  Multiplication=Matrix(K*u)
  Integrator : Integrator
  Signal Specification : SignalSpecification  Dimensions=[size(C,1) 1]
  Sum : Sum  Inputs=+++
  xhat : Outport
  wires:
  Add1/1 -> Signal Specification/1
  Integrator/1 -> Gain3/1, xhat/1, Gain1/1
  Gain1/1 -> Add1/1
  Sum/1 -> Integrator/1
  y/1 -> Add1/2
  u/1 -> Gain/1
  Gain/1 -> Sum/3
  Gain3/1 -> Sum/2
  Signal Specification/1 -> Gain2/1
  Gain2/1 -> Sum/1

== system lc_state_fb_obs_estStatesR/Vehicle5/Input Filter ==
  In1 : Inport
  Demux : Demux
  Mux1 : Mux
  Transfer Fcn{,1..3} (4 alike) : TransferFcn  Denominator=[inputTau 1]
  Out1 : Outport
  wires:
  Demux/1 -> Transfer Fcn/1
  Demux/2 -> Transfer Fcn1/1
  Demux/3 -> Transfer Fcn2/1
  In1/1 -> Demux/1
  Demux/4 -> Transfer Fcn3/1
  Mux1/1 -> Out1/1
  Transfer Fcn/1 -> Mux1/1
  Transfer Fcn1/1 -> Mux1/2
  Transfer Fcn2/1 -> Mux1/3
  Transfer Fcn3/1 -> Mux1/4
